simulink model "hydraulic_ex3"  (R2015b)
settings: Solver=ode23t  StartTime=0.0  StopTime=5  RelTol=1e-3
values from neighbouring files (symbols this model uses):
  A = [-df/m Am/m -Am/m ... (first row only)    [Velocity_ctrl_HYDRAULIC.m]
  A1 = Am    (= 0.00180641577581)    [Velocity_ctrl_HYDRAULIC.m]
  A2 = Am    (= 0.00180641577581)    [Velocity_ctrl_HYDRAULIC.m]
  B = [ 0 -1/m ... (first row only)    [Velocity_ctrl_HYDRAULIC.m]
  C = [1 0 0; 0 1 0; 0 0 1]    [Velocity_ctrl_HYDRAULIC.m]
  Cf = Volume0/B    (= 6.87223392973e-13)    [Velocity_ctrl_HYDRAULIC.m]
  D = [0 0; 0 0; 0 0]    [Velocity_ctrl_HYDRAULIC.m]    (also in ex1.m = 0; position_ctrl.m = (2*J^2*zeta*omega*omega2*r^2+J^2*omega^2*r^2-2*J*zeta*d*omeg; velocity_ctrl.m = 0)
  df = uf    (= 200)    [Velocity_ctrl_HYDRAULIC.m]
  Fe = 10000    [Velocity_ctrl_HYDRAULIC.m]
  m = 100    [Velocity_ctrl_HYDRAULIC.m]    (also in discrete_velocity.m = motor_pars; pcontrol.m = motor_pars; pcontrol_position.m = motor_pars; pdcontroller_position.m = motor_pars)
  p10 = double(solution.p1)    [Velocity_ctrl_HYDRAULIC.m]
  p20 = double(solution.p2)    [Velocity_ctrl_HYDRAULIC.m]
  Ps = 20e6    (= 20000000)    [Velocity_ctrl_HYDRAULIC.m]
  Rv = 1e-4    (= 0.0001)    [Velocity_ctrl_HYDRAULIC.m]
  Tforce = 1    [Velocity_ctrl_HYDRAULIC.m]
  xv = 0.01    [Velocity_ctrl_HYDRAULIC.m]
settings Model: Creator=gabri  LastModifiedBy=andfr

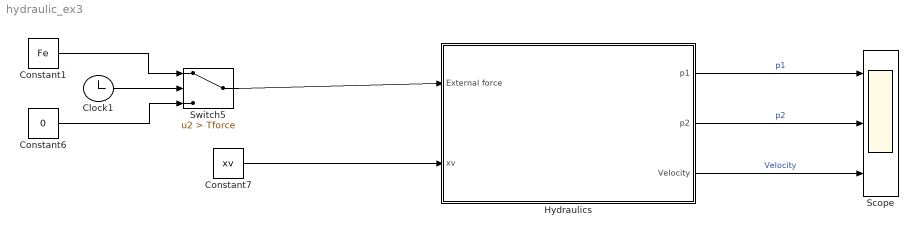
== system hydraulic_ex3 ==
  Clock1 : Clock
  Constant1 : Constant  Value=Fe
  Constant6 : Constant  Value=0
  Constant7 : Constant  Value=xv
  "Hydraulics " : Subsystem
  Scope : Scope  NumInputPorts=3
  Switch5 : Switch  Criteria=u2 > Threshold  Threshold=Tforce
  wires:
  Clock1/1 -> Switch5/2
  Constant1/1 -> Switch5/1
  Constant6/1 -> Switch5/3
  Switch5/1 -> "Hydraulics "/1(External force)
  Constant7/1 -> "Hydraulics "/2(xv)
  "Hydraulics "/1(p1) -> Scope/1  "p1"
  "Hydraulics "/2(p2) -> Scope/2  "p2"
  "Hydraulics "/3(Velocity) -> Scope/3  "Velocity"

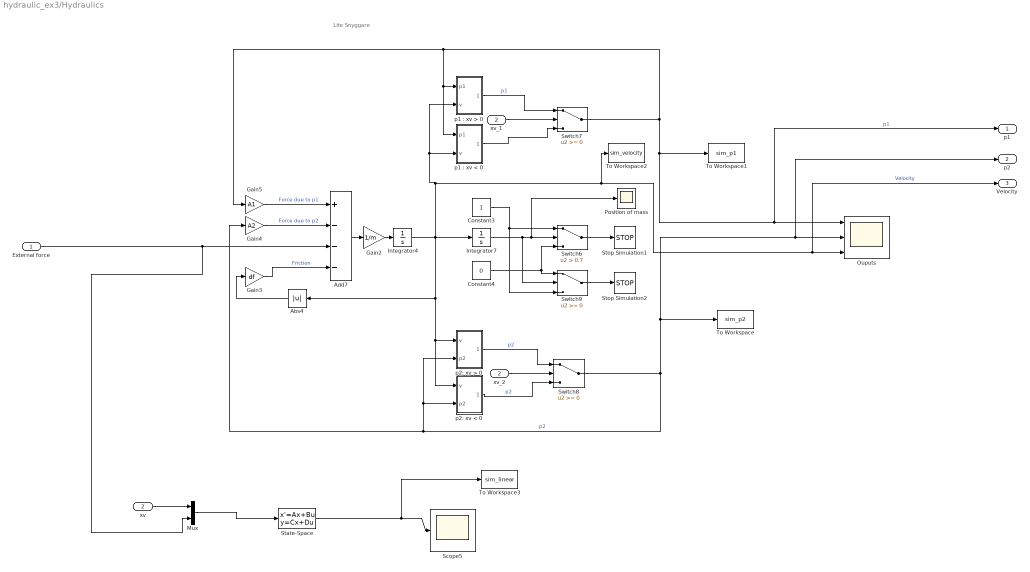
== system hydraulic_ex3/Hydraulics  ==
  note: Lite Snyggare
  External force : Inport
  xv : Inport  Port=2
  Abs4 : Abs
  Add7 : Sum  Inputs=+---
  Constant3 : Constant
  Constant4 : Constant  Value=0
  Gain2 : Gain  Gain=1/m
  Gain3 : Gain  Gain=df
  Gain4 : Gain  Gain=A2
  Gain5 : Gain  Gain=A1
  Integrator4 : Integrator
  Integrator7 : Integrator  InitialCondition=0.35
  Mux : Mux  Inputs=2
  Ouputs : Scope  NumInputPorts=3
  Position of mass : Scope
  Scope5 : Scope
  State-Space : StateSpace  A=A  B=B  C=C  D=D  X0=0
  Stop Simulation1 : Stop
  Stop Simulation2 : Stop
  Switch6 : Switch  Criteria=u2 > Threshold  Threshold=0.7
  Switch7 : Switch
  Switch8 : Switch
  Switch9 : Switch
  To Workspace : ToWorkspace  VariableName=sim_p2  SaveFormat=Timeseries  SampleTime=-1
  To Workspace1 : ToWorkspace  VariableName=sim_p1  SaveFormat=Timeseries  SampleTime=-1
  To Workspace2 : ToWorkspace  VariableName=sim_velocity  SaveFormat=Timeseries  SampleTime=-1
  To Workspace3 : ToWorkspace  VariableName=sim_linear  SaveFormat=Timeseries  SampleTime=-1
  "p1 : xv < 0" : Subsystem
  "p1 : xv > 0" : Subsystem
  p2: xv < 0 : Subsystem
  "p2: xv > 0 " : Subsystem
  xv_1 : InportShadow  Port=2
  xv_2 : InportShadow  Port=2
  p1 : Outport
  p2 : Outport  Port=2
  Velocity : Outport  Port=3
  wires:
  Switch7/1 -> "p1 : xv > 0"/1("p1 "), "p1 : xv < 0"/1(p1), Gain5/1, p1/1, Ouputs/1, To Workspace1/1  "p1"
  Gain2/1 -> Integrator4/1
  xv_2/1 -> Switch8/2
  Mux/1 -> State-Space/1
  Constant3/1 -> Switch9/3, Switch6/1
  "p1 : xv > 0"/1(Out1) -> Switch7/1  "p1"
  Add7/1 -> Gain2/1
  Integrator7/1 -> Switch9/2, Position of mass/1, Switch6/2
  xv/1 -> Mux/1
  Switch8/1 -> p2: xv < 0/2(p2), "p2: xv > 0 "/2(p2), Gain4/1, p2/1, Ouputs/2, To Workspace/1  "p2"
  External force/1 -> Mux/2, Add7/3
  "p2: xv > 0 "/1(Out1) -> Switch8/1  "p2"
  xv_1/1 -> Switch7/2
  Integrator4/1 -> Integrator7/1, "p1 : xv < 0"/2(v), "p1 : xv > 0"/2(v), Velocity/1, Ouputs/3, To Workspace2/1, Abs4/1, "p2: xv > 0 "/1(v), p2: xv < 0/1(v)  "Velocity"
  Abs4/1 -> Gain3/1
  Gain3/1 -> Add7/4  "Friction"
  Gain5/1 -> Add7/1  "Force due to p1"
  Switch9/1 -> Stop Simulation2/1
  State-Space/1 -> To Workspace3/1, Scope5/1
  Switch6/1 -> Stop Simulation1/1
  "p1 : xv < 0"/1(Out1) -> Switch7/3
  p2: xv < 0/1(Out1) -> Switch8/3  "p2"
  Constant4/1 -> Switch6/3, Switch9/1
  Gain4/1 -> Add7/2  "Force due to p2"

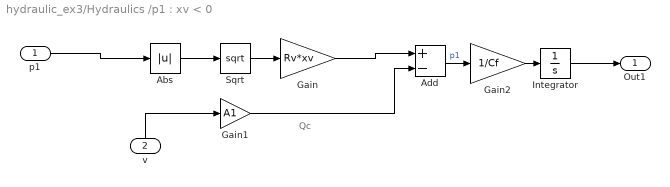
== system hydraulic_ex3/Hydraulics /p1 : xv < 0 ==
  note: Qc
  p1 : Inport
  v : Inport  Port=2
  Abs : Abs
  Add : Sum  Inputs=+-
  Gain : Gain  Gain=Rv*xv
  Gain1 : Gain  Gain=A1
  Gain2 : Gain  Gain=1/Cf
  Integrator : Integrator
  Sqrt : Sqrt  SaturateOnIntegerOverflow=on
  Out1 : Outport
  wires:
  v/1 -> Gain1/1
  Gain1/1 -> Add/2
  Abs/1 -> Sqrt/1
  p1/1 -> Abs/1
  Add/1 -> Gain2/1  "p1"
  Gain2/1 -> Integrator/1
  Integrator/1 -> Out1/1
  Sqrt/1 -> Gain/1
  Gain/1 -> Add/1

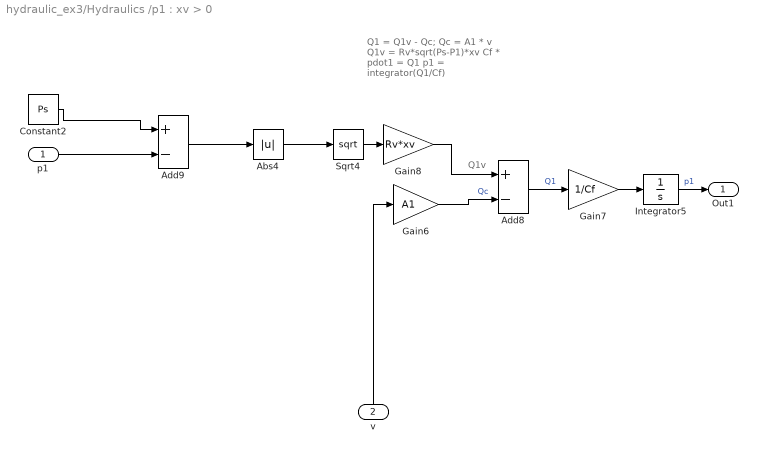
== system hydraulic_ex3/Hydraulics /p1 : xv > 0 ==
  note: Q1v
  note: Q1 = Q1v - Qc;
      | Qc = A1 * v
      | Q1v = Rv*sqrt(Ps-P1)*xv
      | Cf * pdot1 = Q1
      | p1 = integrator(Q1/Cf)
  "p1 " : Inport
  v : Inport  Port=2
  Abs4 : Abs
  Add8 : Sum  Inputs=+-
  Add9 : Sum  Inputs=+-
  Constant2 : Constant  Value=Ps
  Gain6 : Gain  Gain=A1
  Gain7 : Gain  Gain=1/Cf
  Gain8 : Gain  Gain=Rv*xv
  Integrator5 : Integrator  InitialCondition=p10
  Sqrt4 : Sqrt  SaturateOnIntegerOverflow=on
  Out1 : Outport
  wires:
  Add9/1 -> Abs4/1
  Constant2/1 -> Add9/1
  Abs4/1 -> Sqrt4/1
  Gain7/1 -> Integrator5/1
  Gain6/1 -> Add8/2  "Qc"
  Integrator5/1 -> Out1/1  "p1"
  Add8/1 -> Gain7/1  "Q1"
  Sqrt4/1 -> Gain8/1
  Gain8/1 -> Add8/1
  v/1 -> Gain6/1
  "p1 "/1 -> Add9/2

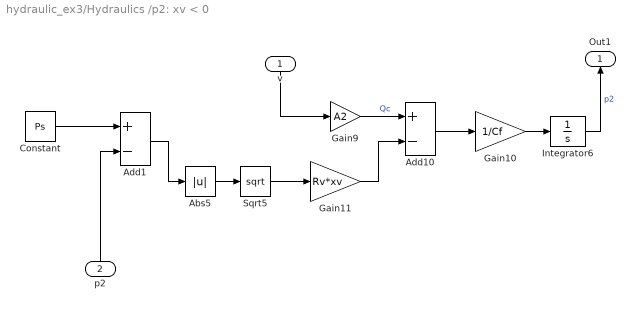
== system hydraulic_ex3/Hydraulics /p2: xv < 0 ==
  v : Inport
  p2 : Inport  Port=2
  Abs5 : Abs
  Add1 : Sum  Inputs=+-
  Add10 : Sum  Inputs=+-
  Constant : Constant  Value=Ps
  Gain10 : Gain  Gain=1/Cf
  Gain11 : Gain  Gain=Rv*xv
  Gain9 : Gain  Gain=A2
  Integrator6 : Integrator
  Sqrt5 : Sqrt  SaturateOnIntegerOverflow=on
  Out1 : Outport
  wires:
  Abs5/1 -> Sqrt5/1
  Gain9/1 -> Add10/1  "Qc"
  Sqrt5/1 -> Gain11/1
  Gain10/1 -> Integrator6/1
  Add10/1 -> Gain10/1
  Integrator6/1 -> Out1/1  "p2"
  v/1 -> Gain9/1
  p2/1 -> Add1/2
  Add1/1 -> Abs5/1
  Constant/1 -> Add1/1
  Gain11/1 -> Add10/2

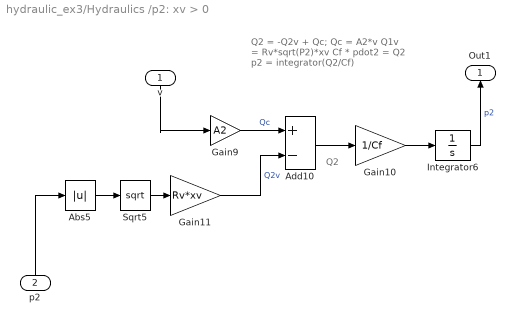
== system hydraulic_ex3/Hydraulics /p2: xv > 0  ==
  note: Q2
  note: Q2 = -Q2v + Qc;
      | Qc = A2*v
      | Q1v = Rv*sqrt(P2)*xv
      | Cf * pdot2 = Q2
      | p2 = integrator(Q2/Cf)
  v : Inport
  p2 : Inport  Port=2
  Abs5 : Abs
  Add10 : Sum  Inputs=+-
  Gain10 : Gain  Gain=1/Cf
  Gain11 : Gain  Gain=Rv*xv
  Gain9 : Gain  Gain=A2
  Integrator6 : Integrator  InitialCondition=p20
  Sqrt5 : Sqrt  SaturateOnIntegerOverflow=on
  Out1 : Outport
  wires:
  p2/1 -> Abs5/1
  v/1 -> Gain9/1
  Integrator6/1 -> Out1/1  "p2"
  Add10/1 -> Gain10/1
  Gain10/1 -> Integrator6/1
  Sqrt5/1 -> Gain11/1
  Gain11/1 -> Add10/2  "Q2v"
  Gain9/1 -> Add10/1  "Qc"
  Abs5/1 -> Sqrt5/1
